simulink model "sousMarin_"  (R2021a)
settings: Solver=VariableStepAuto  StartTime=0.0  StopTime=3000  RelTol=1e-3
values from neighbouring files (symbols this model uses):
  BAT_AUTONOMY_S = BAT_AUTONOMY_H * 3600    (= 72000)    [init_values.m]
  INIT_NIV_BAT = 50    [init_values.m]
  SIMU_ACCEL = 10    [init_values.m]
  TIME_APPEL_CHARGE_S = TIME_APPEL_CHARGE_M * 60    (= 3600)    [init_values.m]
  TIME_PHOTO_S = 4    [init_values.m]
  TIME_TO_CHARGE_S = TIME_TO_CHARGE_M*60    (= 3000)    [init_values.m]
  VARIANCE_INCL_FOND = 25    [init_values.m]
  VITESSE_MAX_MS = 0.5    [init_values.m]
libraries: pid_lib x3, simulink_extras x2, simulink x1, truetime x1
settings Model: SimulationMode=accelerator  Creator=jelefl  LastModifiedBy=yamouh
settings SolverCC: AlgebraicLoopSolver=TrustRegion
settings DebuggingCC: SFMachineParentedDataDiag=warning

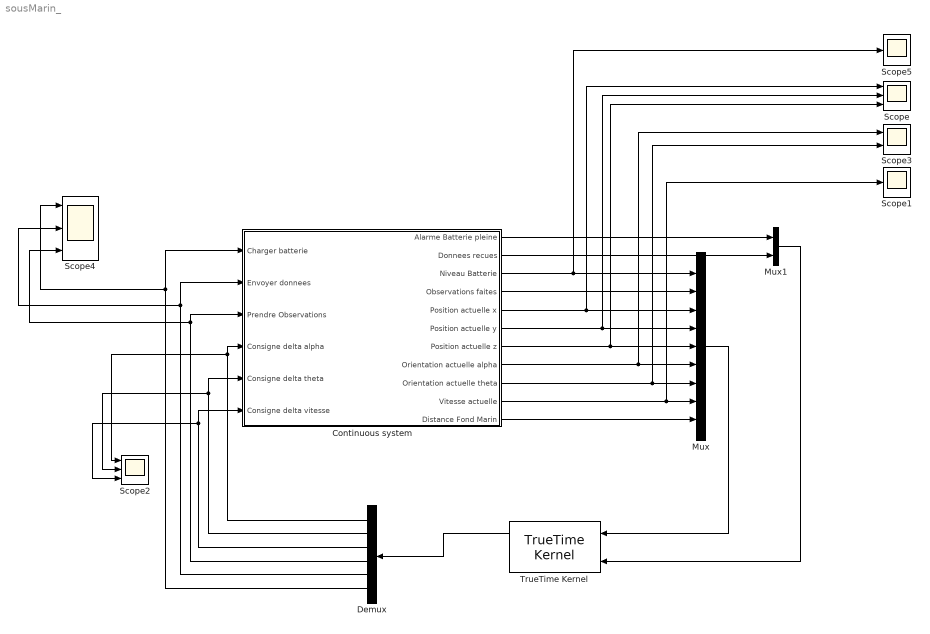
== system sousMarin_ ==
  Continuous system : Subsystem
  Demux : Demux  Outputs=6
  Mux : Mux  Inputs=9
  Mux1 : Mux  Inputs=2
  Scope : Scope  NumInputPorts=3
  Scope1 : Scope
  Scope2 : Scope  NumInputPorts=3
  Scope3 : Scope  NumInputPorts=2
  Scope4 : Scope  NumInputPorts=3
  Scope5 : Scope
  TrueTime Kernel : truetime/TrueTime Kernel  sfun=ctrlSM  args=[]  ninputsoutputs=[9 6]  ntriggers=2  trigtype=falling  nwnodenbr=[]  clockoffsetdrift=[0 0]  schedoutput=on  battery=off  poweroutput=off
  wires:
  Continuous system/3(Niveau Batterie) -> Scope5/1, Mux/1
  Continuous system/5(Position actuelle x) -> Scope/1, Mux/3
  Continuous system/6(Position actuelle y) -> Scope/2, Mux/4
  Continuous system/7(Position actuelle z) -> Scope/3, Mux/5
  Continuous system/8(Orientation actuelle alpha) -> Mux/6, Scope3/1
  Continuous system/9(Orientation actuelle theta) -> Mux/7, Scope3/2
  Mux/1 -> TrueTime Kernel/1
  TrueTime Kernel/1 -> Demux/1
  Demux/2 -> Scope2/2, Continuous system/5(Consigne delta theta)
  Demux/3 -> Scope2/3, Continuous system/6(Consigne delta vitesse)
  Demux/1 -> Scope2/1, Continuous system/4(Consigne delta alpha)
  Continuous system/10(Vitesse actuelle) -> Mux/8, Scope1/1
  Continuous system/11(Distance Fond Marin) -> Mux/9
  Continuous system/4(Observations faites) -> Mux/2
  Continuous system/1(Alarme Batterie pleine) -> Mux1/1
  Continuous system/2(Donnees recues) -> Mux1/2
  Demux/4 -> Scope4/3, Continuous system/3(Prendre Observations)
  Demux/5 -> Continuous system/2(Envoyer donnees), Scope4/2
  Demux/6 -> Continuous system/1(Charger batterie), Scope4/1
  Mux1/1 -> TrueTime Kernel/2

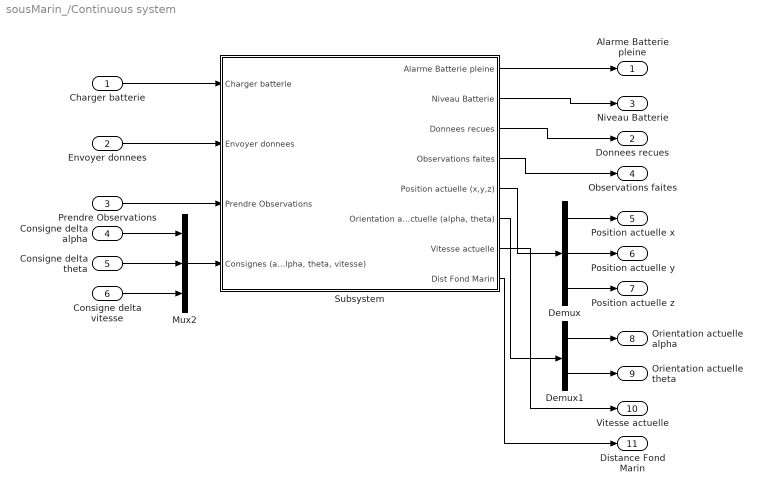
== system sousMarin_/Continuous system ==
  Charger batterie : Inport
  Envoyer donnees : Inport  Port=2
  Prendre Observations : Inport  Port=3
  Consigne delta alpha : Inport  Port=4
  Consigne delta theta : Inport  Port=5
  Consigne delta vitesse : Inport  Port=6
  Demux : Demux  Outputs=3
  Demux1 : Demux  Outputs=2
  Mux2 : Mux  Inputs=3
  Subsystem : Subsystem
  Alarme Batterie pleine : Outport  VectorParamsAs1DForOutWhenUnconnected=off
  Donnees recues : Outport  Port=2  VectorParamsAs1DForOutWhenUnconnected=off
  Niveau Batterie : Outport  Port=3  VectorParamsAs1DForOutWhenUnconnected=off
  Observations faites : Outport  Port=4  VectorParamsAs1DForOutWhenUnconnected=off
  Position actuelle x : Outport  Port=5  VectorParamsAs1DForOutWhenUnconnected=off
  Position actuelle y : Outport  Port=6  VectorParamsAs1DForOutWhenUnconnected=off
  Position actuelle z : Outport  Port=7  VectorParamsAs1DForOutWhenUnconnected=off
  Orientation actuelle alpha : Outport  Port=8  VectorParamsAs1DForOutWhenUnconnected=off
  Orientation actuelle theta : Outport  Port=9  VectorParamsAs1DForOutWhenUnconnected=off
  Vitesse actuelle : Outport  Port=10  VectorParamsAs1DForOutWhenUnconnected=off
  Distance Fond Marin : Outport  Port=11  VectorParamsAs1DForOutWhenUnconnected=off
  wires:
  Prendre Observations/1 -> Subsystem/3(Prendre Observations)
  Envoyer donnees/1 -> Subsystem/2(Envoyer donnees)
  Charger batterie/1 -> Subsystem/1(Charger batterie)
  Mux2/1 -> Subsystem/4("Consignes (alpha, theta, vitesse)")
  Consigne delta alpha/1 -> Mux2/1
  Consigne delta theta/1 -> Mux2/2
  Consigne delta vitesse/1 -> Mux2/3
  Subsystem/1(Alarme Batterie pleine) -> Alarme Batterie pleine/1
  Subsystem/2(Niveau Batterie) -> Niveau Batterie/1
  Subsystem/3(Donnees recues) -> Donnees recues/1
  Subsystem/4(Observations faites) -> Observations faites/1
  Subsystem/5(Position actuelle (x,y,z)) -> Demux/1
  Demux/1 -> Position actuelle x/1
  Demux/2 -> Position actuelle y/1
  Demux/3 -> Position actuelle z/1
  Demux1/1 -> Orientation actuelle alpha/1
  Demux1/2 -> Orientation actuelle theta/1
  Subsystem/6("Orientation actuelle (alpha, theta)") -> Demux1/1
  Subsystem/7(Vitesse actuelle) -> Vitesse actuelle/1
  Subsystem/8(Dist Fond Marin) -> Distance Fond Marin/1

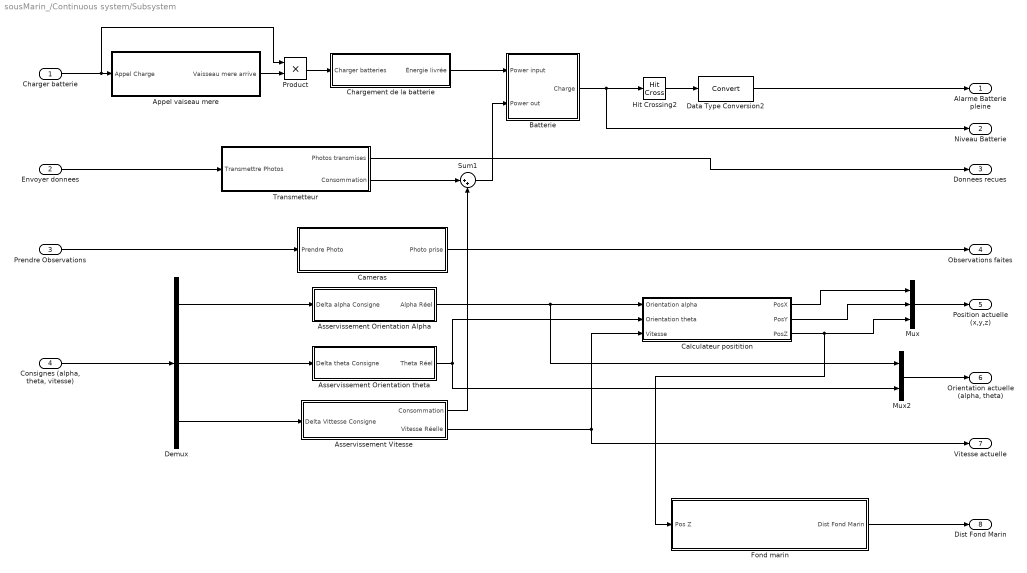
== system sousMarin_/Continuous system/Subsystem ==
  Charger batterie : Inport
  Envoyer donnees : Inport  Port=2
  Prendre Observations : Inport  Port=3
  "Consignes (alpha, theta, vitesse)" : Inport  Port=4
  Appel vaiseau mere : Subsystem
  Asservissement Orientation Alpha : Subsystem
  Asservissement Orientation theta : Subsystem
  Asservissement Vitesse : Subsystem
  Batterie : Subsystem
  Calculateur positition : Subsystem
  Cameras : Subsystem
  Chargement de la batterie : Subsystem
  Data Type Conversion2 : DataTypeConversion
  Demux : Demux  Outputs=3
  Fond marin : Subsystem
  Hit Crossing2 : HitCross  HitCrossingOffset=99.99  HitCrossingDirection=rising
  Mux : Mux  Inputs=3
  Mux2 : Mux  Inputs=2
  Product : Product
  Sum1 : Sum  Inputs=|++
  Transmetteur : Subsystem
  Alarme Batterie pleine : Outport  VectorParamsAs1DForOutWhenUnconnected=off
  Niveau Batterie : Outport  Port=2  VectorParamsAs1DForOutWhenUnconnected=off
  Donnees recues : Outport  Port=3  VectorParamsAs1DForOutWhenUnconnected=off
  Observations faites : Outport  Port=4  VectorParamsAs1DForOutWhenUnconnected=off
  Position actuelle (x,y,z) : Outport  Port=5  VectorParamsAs1DForOutWhenUnconnected=off
  "Orientation actuelle (alpha, theta)" : Outport  Port=6  VectorParamsAs1DForOutWhenUnconnected=off
  Vitesse actuelle : Outport  Port=7  VectorParamsAs1DForOutWhenUnconnected=off
  Dist Fond Marin : Outport  Port=8  VectorParamsAs1DForOutWhenUnconnected=off
  wires:
  Batterie/1(Charge) -> Niveau Batterie/1, Hit Crossing2/1
  Hit Crossing2/1 -> Data Type Conversion2/1
  Data Type Conversion2/1 -> Alarme Batterie pleine/1
  Calculateur positition/3(PosZ) -> Fond marin/1(Pos Z), Mux/3
  Prendre Observations/1 -> Cameras/1(Prendre Photo)
  Transmetteur/1(Photos transmises) -> Donnees recues/1
  Cameras/1(Photo prise) -> Observations faites/1
  Asservissement Vitesse/2(Vitesse Réelle) -> Calculateur positition/3(Vitesse), Vitesse actuelle/1
  Calculateur positition/2(PosY) -> Mux/2
  Calculateur positition/1(PosX) -> Mux/1
  Mux/1 -> Position actuelle (x,y,z)/1
  Chargement de la batterie/1(Énergie livrée) -> Batterie/1(Power input)
  Asservissement Orientation Alpha/1(Alpha Réel) -> Mux2/1, Calculateur positition/1(Orientation alpha)
  Envoyer donnees/1 -> Transmetteur/1(Transmettre Photos)
  Appel vaiseau mere/1(Vaisseau mere arrive) -> Product/2
  Product/1 -> Chargement de la batterie/1(Charger batteries)
  Charger batterie/1 -> Product/1, Appel vaiseau mere/1(Appel Charge)
  Asservissement Orientation theta/1(Theta Réel) -> Calculateur positition/2(Orientation theta), Mux2/2
  Sum1/1 -> Batterie/2(Power out)
  Transmetteur/2(Consommation) -> Sum1/1
  Asservissement Vitesse/1(Consommation) -> Sum1/2
  Demux/2 -> Asservissement Orientation theta/1(Delta theta Consigne)
  Demux/3 -> Asservissement Vitesse/1(Delta Vittesse Consigne)
  Demux/1 -> Asservissement Orientation Alpha/1(Delta alpha Consigne)
  "Consignes (alpha, theta, vitesse)"/1 -> Demux/1
  Mux2/1 -> "Orientation actuelle (alpha, theta)"/1
  Fond marin/1(Dist Fond Marin) -> Dist Fond Marin/1

== system sousMarin_/Continuous system/Subsystem/Appel vaiseau mere ==
  Appel Charge : Inport
  Vaisseau mere en deplacement : Subsystem  TreatAsAtomicUnit=on
  Vaisseau mere arrive : Outport  VectorParamsAs1DForOutWhenUnconnected=off
  wires:
  Vaisseau mere en deplacement/1(Vaisseau mere arrive) -> Vaisseau mere arrive/1
  Appel Charge/1 -> Vaisseau mere en deplacement/Reset

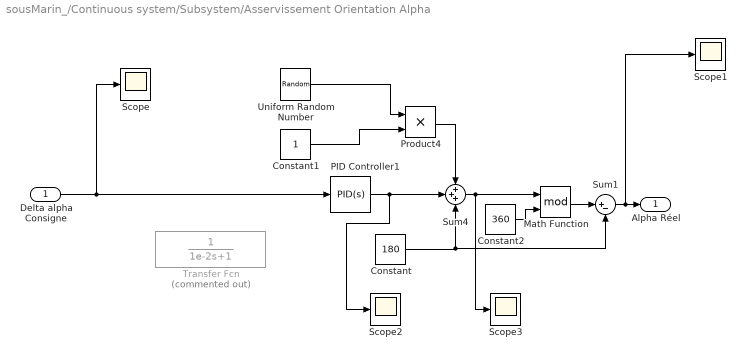
== system sousMarin_/Continuous system/Subsystem/Asservissement Orientation Alpha ==
  Delta alpha Consigne : Inport
  Constant : Constant  Value=180
  Constant1 : Constant
  Constant2 : Constant  Value=360
  Math Function : Math  Operator=mod  SaturateOnIntegerOverflow=on
  PID Controller1 : pid_lib/PID Controller  Controller=PID  Form=Parallel  TimeDomain=Continuous-time  UseExternalTs=off  SampleTime=-1  IntegratorMethod=Forward Euler  FilterMethod=Forward Euler  ControllerParametersSource=internal  P=.1  I=5  D=0  UseFilter=on  N=0.1  TunerSelectOption=Transfer Function Based (PID Tuner App)  InitialConditionSource=internal  InitialConditionForIntegrator=0  InitialConditionForFilter=0  DifferentiatorICPrevScaledInput=0  ExternalReset=none  TrackingMode=off  Kt=1  LimitOutput=off  SatLimitsSource=internal  UpperSaturationLimit=inf  LowerSaturationLimit=-inf  LinearizeAsGain=on  AntiWindupMode=none  Kb=1  POutMin=[]  POutMax=[]  IOutMin=[]  IOutMax=[]  DOutMin=[]  DOutMax=[]  NOutMin=[]  NOutMax=[]  SumOutMin=[]  SumOutMax=[]  SaturationOutMin=[]  SaturationOutMax=[]  PParamMin=[]  PParamMax=[]  IParamMin=[]  IParamMax=[]  DParamMin=[]  DParamMax=[]  NParamMin=[]  NParamMax=[]  KbParamMin=[]  KbParamMax=[]  KtParamMin=[]  KtParamMax=[]  KbOutMin=[]  KbOutMax=[]  KtOutMin=[]  KtOutMax=[]  IntegratorOutMin=[]  IntegratorOutMax=[]  FilterOutMin=[]  FilterOutMax=[]  SumI1OutMin=[]  SumI1OutMax=[]  SumI2OutMin=[]  SumI2OutMax=[]  SumI3OutMin=[]  SumI3OutMax=[]  SumI4OutMin=[]  SumI4OutMax=[]  SumDOutMin=[]  SumDOutMax=[]  DifferentiatorOutMin=[]  DifferentiatorOutMax=[]  FilterDiffOutCoefMin=[]  FilterDiffOutCoefMax=[]  ReciprocalOutMin=[]  ReciprocalOutMax=[]  SumDenOutMin=[]  SumDenOutMax=[]  SumNumOutMin=[]  SumNumOutMax=[]  DivideOutMin=[]  DivideOutMax=[]  UdiffTsProdOutMin=[]  UdiffTsProdOutMax=[]  NTsProdOutMin=[]  NTsProdOutMax=[]  UintegralTsProdOutMin=[]  UintegralTsProdOutMax=[]  UngainTsProdOutMin=[]  UngainTsProdOutMax=[]  IntegratorContinuousStateAttributes=''  IntegratorStateMustResolveToSignalObject=off  IntegratorRTWStateStorageClass=Auto  FilterContinuousStateAttributes=''  FilterStateMustResolveToSignalObject=off  FilterRTWStateStorageClass=Auto  ParallelPVariant=InternalParameters  IdealPVariant=Disabled  IVariant=InternalParameters  DVariant=InternalParameters  IntegratorVariant=Continuous  SatVariant=Disabled  AWVariant=Passthrough  PCopyVariant=Disabled  TRVariant=Disabled  FdbkBlocksVariant=Forward  IdealPFdbkVariant=Disabled  SatFdbkVariant=Disabled  DerivativeFilterVariant=ContFilter  NVariant=InternalParameters  NCopyVariant=Disabled  FilterICVariant=InternalICsFilter  IntegratorICVariant=InternalICs  ExternalResetVariant=Disabled  TRSumVariant=Passthrough  SumFdbkVariant=Disabled  SumVariant=Sum_PID  TsampFilterVariant=InternalTs  TsampNgainVariant=Passthrough  TsampIntegralVariant=Passthrough  ExternalSaturationOutDataTypeStr=Inherit: Same as second input
  Product4 : Product
  Scope{,1..3} (4 alike) : Scope
  Sum1 : Sum  Inputs=|+-
  Sum4 : Sum  Inputs=+++
  Transfer Fcn : TransferFcn  Commented=on  Denominator=[1e-2 1]
  Uniform Random Number : UniformRandomNumber  SampleTime=0.1
  Alpha Réel : Outport  VectorParamsAs1DForOutWhenUnconnected=off
  wires:
  Product4/1 -> Sum4/1
  Uniform Random Number/1 -> Product4/1
  Constant1/1 -> Product4/2
  PID Controller1/1 -> Scope2/1, Sum4/2
  Delta alpha Consigne/1 -> PID Controller1/1, Scope/1
  Constant/1 -> Sum4/3, Sum1/2
  Math Function/1 -> Sum1/1
  Constant2/1 -> Math Function/2
  Sum1/1 -> Scope1/1, Alpha Réel/1
  Sum4/1 -> Scope3/1, Math Function/1

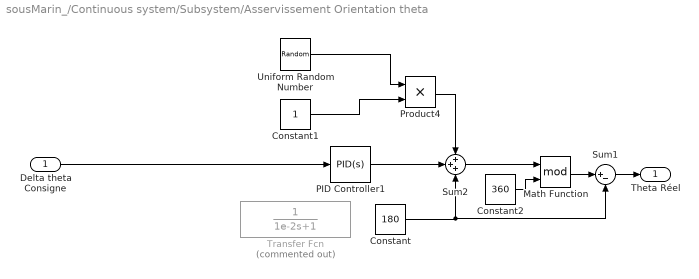
== system sousMarin_/Continuous system/Subsystem/Asservissement Orientation theta ==
  Delta theta Consigne : Inport
  Constant : Constant  Value=180
  Constant1 : Constant
  Constant2 : Constant  Value=360
  Math Function : Math  Operator=mod  SaturateOnIntegerOverflow=on
  PID Controller1 : pid_lib/PID Controller  Controller=PID  Form=Parallel  TimeDomain=Continuous-time  UseExternalTs=off  SampleTime=-1  IntegratorMethod=Forward Euler  FilterMethod=Forward Euler  ControllerParametersSource=internal  P=.1  I=5  D=0  UseFilter=on  N=0.1  TunerSelectOption=Transfer Function Based (PID Tuner App)  InitialConditionSource=internal  InitialConditionForIntegrator=0  InitialConditionForFilter=0  DifferentiatorICPrevScaledInput=0  ExternalReset=none  TrackingMode=off  Kt=1  LimitOutput=off  SatLimitsSource=internal  UpperSaturationLimit=inf  LowerSaturationLimit=-inf  LinearizeAsGain=on  AntiWindupMode=none  Kb=1  POutMin=[]  POutMax=[]  IOutMin=[]  IOutMax=[]  DOutMin=[]  DOutMax=[]  NOutMin=[]  NOutMax=[]  SumOutMin=[]  SumOutMax=[]  SaturationOutMin=[]  SaturationOutMax=[]  PParamMin=[]  PParamMax=[]  IParamMin=[]  IParamMax=[]  DParamMin=[]  DParamMax=[]  NParamMin=[]  NParamMax=[]  KbParamMin=[]  KbParamMax=[]  KtParamMin=[]  KtParamMax=[]  KbOutMin=[]  KbOutMax=[]  KtOutMin=[]  KtOutMax=[]  IntegratorOutMin=[]  IntegratorOutMax=[]  FilterOutMin=[]  FilterOutMax=[]  SumI1OutMin=[]  SumI1OutMax=[]  SumI2OutMin=[]  SumI2OutMax=[]  SumI3OutMin=[]  SumI3OutMax=[]  SumI4OutMin=[]  SumI4OutMax=[]  SumDOutMin=[]  SumDOutMax=[]  DifferentiatorOutMin=[]  DifferentiatorOutMax=[]  FilterDiffOutCoefMin=[]  FilterDiffOutCoefMax=[]  ReciprocalOutMin=[]  ReciprocalOutMax=[]  SumDenOutMin=[]  SumDenOutMax=[]  SumNumOutMin=[]  SumNumOutMax=[]  DivideOutMin=[]  DivideOutMax=[]  UdiffTsProdOutMin=[]  UdiffTsProdOutMax=[]  NTsProdOutMin=[]  NTsProdOutMax=[]  UintegralTsProdOutMin=[]  UintegralTsProdOutMax=[]  UngainTsProdOutMin=[]  UngainTsProdOutMax=[]  IntegratorContinuousStateAttributes=''  IntegratorStateMustResolveToSignalObject=off  IntegratorRTWStateStorageClass=Auto  FilterContinuousStateAttributes=''  FilterStateMustResolveToSignalObject=off  FilterRTWStateStorageClass=Auto  ParallelPVariant=InternalParameters  IdealPVariant=Disabled  IVariant=InternalParameters  DVariant=InternalParameters  IntegratorVariant=Continuous  SatVariant=Disabled  AWVariant=Passthrough  PCopyVariant=Disabled  TRVariant=Disabled  FdbkBlocksVariant=Forward  IdealPFdbkVariant=Disabled  SatFdbkVariant=Disabled  DerivativeFilterVariant=ContFilter  NVariant=InternalParameters  NCopyVariant=Disabled  FilterICVariant=InternalICsFilter  IntegratorICVariant=InternalICs  ExternalResetVariant=Disabled  TRSumVariant=Passthrough  SumFdbkVariant=Disabled  SumVariant=Sum_PID  TsampFilterVariant=InternalTs  TsampNgainVariant=Passthrough  TsampIntegralVariant=Passthrough  ExternalSaturationOutDataTypeStr=Inherit: Same as second input
  Product4 : Product
  Sum1 : Sum  Inputs=|+-
  Sum2 : Sum  Inputs=+++
  Transfer Fcn : TransferFcn  Commented=on  Denominator=[1e-2 1]
  Uniform Random Number : UniformRandomNumber  SampleTime=0.1
  Theta Réel : Outport  VectorParamsAs1DForOutWhenUnconnected=off
  wires:
  Product4/1 -> Sum2/1
  Uniform Random Number/1 -> Product4/1
  Constant1/1 -> Product4/2
  PID Controller1/1 -> Sum2/2
  Delta theta Consigne/1 -> PID Controller1/1
  Sum1/1 -> Theta Réel/1
  Constant/1 -> Sum2/3, Sum1/2
  Constant2/1 -> Math Function/2
  Math Function/1 -> Sum1/1
  Sum2/1 -> Math Function/1

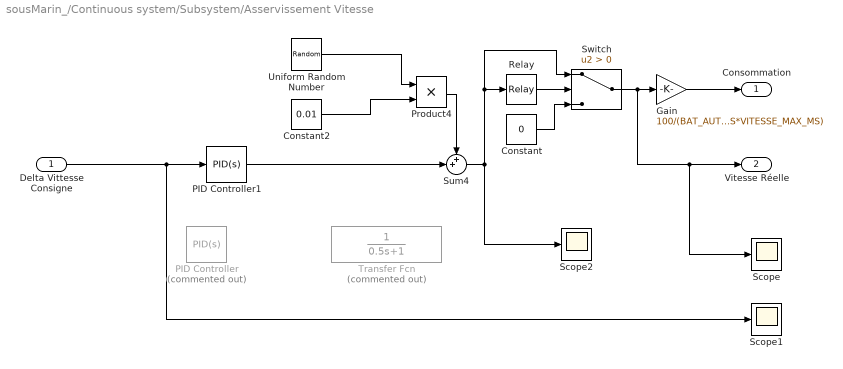
== system sousMarin_/Continuous system/Subsystem/Asservissement Vitesse ==
  Delta Vittesse Consigne : Inport
  Constant : Constant  Value=0
  Constant2 : Constant  Value=0.01
  Gain : Gain  Gain=100/(BAT_AUTONOMY_S*VITESSE_MAX_MS)
  PID Controller : simulink/Continuous/PID Controller  Commented=on  Controller=PID  Form=Parallel  TimeDomain=Continuous-time  UseExternalTs=off  SampleTime=-1  IntegratorMethod=Forward Euler  FilterMethod=Forward Euler  ControllerParametersSource=internal  P=1  I=1  D=0  UseFilter=on  N=100  TunerSelectOption=Transfer Function Based (PID Tuner App)  InitialConditionSource=internal  InitialConditionForIntegrator=0  InitialConditionForFilter=0  DifferentiatorICPrevScaledInput=0  ExternalReset=none  TrackingMode=off  Kt=1  LimitOutput=off  UpperSaturationLimit=inf  LowerSaturationLimit=-inf  LinearizeAsGain=on  AntiWindupMode=none  Kb=1  POutMin=[]  POutMax=[]  IOutMin=[]  IOutMax=[]  DOutMin=[]  DOutMax=[]  NOutMin=[]  NOutMax=[]  SumOutMin=[]  SumOutMax=[]  SaturationOutMin=[]  SaturationOutMax=[]  PParamMin=[]  PParamMax=[]  IParamMin=[]  IParamMax=[]  DParamMin=[]  DParamMax=[]  NParamMin=[]  NParamMax=[]  KbParamMin=[]  KbParamMax=[]  KtParamMin=[]  KtParamMax=[]  KbOutMin=[]  KbOutMax=[]  KtOutMin=[]  KtOutMax=[]  IntegratorOutMin=[]  IntegratorOutMax=[]  FilterOutMin=[]  FilterOutMax=[]  SumI1OutMin=[]  SumI1OutMax=[]  SumI2OutMin=[]  SumI2OutMax=[]  SumI3OutMin=[]  SumI3OutMax=[]  SumI4OutMin=[]  SumI4OutMax=[]  SumDOutMin=[]  SumDOutMax=[]  DifferentiatorOutMin=[]  DifferentiatorOutMax=[]  FilterDiffOutCoefMin=[]  FilterDiffOutCoefMax=[]  ReciprocalOutMin=[]  ReciprocalOutMax=[]  SumDenOutMin=[]  SumDenOutMax=[]  SumNumOutMin=[]  SumNumOutMax=[]  DivideOutMin=[]  DivideOutMax=[]  UdiffTsProdOutMin=[]  UdiffTsProdOutMax=[]  NTsProdOutMin=[]  NTsProdOutMax=[]  UintegralTsProdOutMin=[]  UintegralTsProdOutMax=[]  UngainTsProdOutMin=[]  UngainTsProdOutMax=[]  IntegratorContinuousStateAttributes=''  IntegratorStateMustResolveToSignalObject=off  IntegratorRTWStateStorageClass=Auto  FilterContinuousStateAttributes=''  FilterStateMustResolveToSignalObject=off  FilterRTWStateStorageClass=Auto  ParallelPVariant=InternalParameters  IdealPVariant=Disabled  IVariant=InternalParameters  DVariant=InternalParameters  IntegratorVariant=Continuous  SatVariant=Disabled  AWVariant=Passthrough  PCopyVariant=Disabled  TRVariant=Disabled  FdbkBlocksVariant=Forward  IdealPFdbkVariant=Disabled  SatFdbkVariant=Disabled  DerivativeFilterVariant=ContFilter  NVariant=InternalParameters  NCopyVariant=Disabled  FilterICVariant=InternalICsFilter  IntegratorICVariant=InternalICs  ExternalResetVariant=Disabled  TRSumVariant=Passthrough  SumFdbkVariant=Disabled  SumVariant=Sum_PID  TsampFilterVariant=InternalTs  TsampNgainVariant=Passthrough  TsampIntegralVariant=Passthrough
  PID Controller1 : pid_lib/PID Controller  Controller=PID  Form=Parallel  TimeDomain=Continuous-time  UseExternalTs=off  SampleTime=-1  IntegratorMethod=Forward Euler  FilterMethod=Forward Euler  ControllerParametersSource=internal  P=.1  I=5  D=0  UseFilter=on  N=0.1  TunerSelectOption=Transfer Function Based (PID Tuner App)  InitialConditionSource=internal  InitialConditionForIntegrator=0  InitialConditionForFilter=0  DifferentiatorICPrevScaledInput=0  ExternalReset=none  TrackingMode=off  Kt=1  LimitOutput=off  SatLimitsSource=internal  UpperSaturationLimit=inf  LowerSaturationLimit=-inf  LinearizeAsGain=on  AntiWindupMode=none  Kb=1  POutMin=[]  POutMax=[]  IOutMin=[]  IOutMax=[]  DOutMin=[]  DOutMax=[]  NOutMin=[]  NOutMax=[]  SumOutMin=[]  SumOutMax=[]  SaturationOutMin=[]  SaturationOutMax=[]  PParamMin=[]  PParamMax=[]  IParamMin=[]  IParamMax=[]  DParamMin=[]  DParamMax=[]  NParamMin=[]  NParamMax=[]  KbParamMin=[]  KbParamMax=[]  KtParamMin=[]  KtParamMax=[]  KbOutMin=[]  KbOutMax=[]  KtOutMin=[]  KtOutMax=[]  IntegratorOutMin=[]  IntegratorOutMax=[]  FilterOutMin=[]  FilterOutMax=[]  SumI1OutMin=[]  SumI1OutMax=[]  SumI2OutMin=[]  SumI2OutMax=[]  SumI3OutMin=[]  SumI3OutMax=[]  SumI4OutMin=[]  SumI4OutMax=[]  SumDOutMin=[]  SumDOutMax=[]  DifferentiatorOutMin=[]  DifferentiatorOutMax=[]  FilterDiffOutCoefMin=[]  FilterDiffOutCoefMax=[]  ReciprocalOutMin=[]  ReciprocalOutMax=[]  SumDenOutMin=[]  SumDenOutMax=[]  SumNumOutMin=[]  SumNumOutMax=[]  DivideOutMin=[]  DivideOutMax=[]  UdiffTsProdOutMin=[]  UdiffTsProdOutMax=[]  NTsProdOutMin=[]  NTsProdOutMax=[]  UintegralTsProdOutMin=[]  UintegralTsProdOutMax=[]  UngainTsProdOutMin=[]  UngainTsProdOutMax=[]  IntegratorContinuousStateAttributes=''  IntegratorStateMustResolveToSignalObject=off  IntegratorRTWStateStorageClass=Auto  FilterContinuousStateAttributes=''  FilterStateMustResolveToSignalObject=off  FilterRTWStateStorageClass=Auto  ParallelPVariant=InternalParameters  IdealPVariant=Disabled  IVariant=InternalParameters  DVariant=InternalParameters  IntegratorVariant=Continuous  SatVariant=Disabled  AWVariant=Passthrough  PCopyVariant=Disabled  TRVariant=Disabled  FdbkBlocksVariant=Forward  IdealPFdbkVariant=Disabled  SatFdbkVariant=Disabled  DerivativeFilterVariant=ContFilter  NVariant=InternalParameters  NCopyVariant=Disabled  FilterICVariant=InternalICsFilter  IntegratorICVariant=InternalICs  ExternalResetVariant=Disabled  TRSumVariant=Passthrough  SumFdbkVariant=Disabled  SumVariant=Sum_PID  TsampFilterVariant=InternalTs  TsampNgainVariant=Passthrough  TsampIntegralVariant=Passthrough  ExternalSaturationOutDataTypeStr=Inherit: Same as second input
  Product4 : Product
  Relay : Relay  OnSwitchValue=0.011  OffSwitchValue=0.01
  Scope : Scope
  Scope1 : Scope
  Scope2 : Scope
  Sum4 : Sum  Inputs=++|
  Switch : Switch  Criteria=u2 > Threshold
  Transfer Fcn : TransferFcn  Commented=on  Denominator=[0.5 1]
  Uniform Random Number : UniformRandomNumber  SampleTime=0.1
  Consommation : Outport  VectorParamsAs1DForOutWhenUnconnected=off
  Vitesse Réelle : Outport  Port=2  VectorParamsAs1DForOutWhenUnconnected=off
  wires:
  Sum4/1 -> Switch/1, Relay/1, Scope2/1
  Relay/1 -> Switch/2
  Gain/1 -> Consommation/1
  Constant/1 -> Switch/3
  Uniform Random Number/1 -> Product4/1
  Constant2/1 -> Product4/2
  Product4/1 -> Sum4/1
  Delta Vittesse Consigne/1 -> Scope1/1, PID Controller1/1
  PID Controller1/1 -> Sum4/2
  Switch/1 -> Scope/1, Vitesse Réelle/1, Gain/1

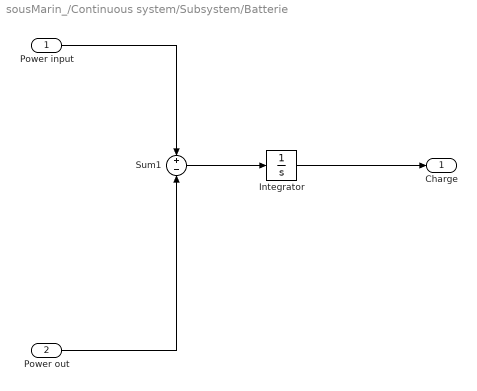
== system sousMarin_/Continuous system/Subsystem/Batterie ==
  Power input : Inport
  Power out : Inport  Port=2
  Integrator : Integrator  InitialCondition=INIT_NIV_BAT  LimitOutput=on  UpperSaturationLimit=100  LowerSaturationLimit=0
  Sum1 : Sum  Inputs=+-
  Charge : Outport  VectorParamsAs1DForOutWhenUnconnected=off
  wires:
  Sum1/1 -> Integrator/1
  Power input/1 -> Sum1/1
  Power out/1 -> Sum1/2
  Integrator/1 -> Charge/1

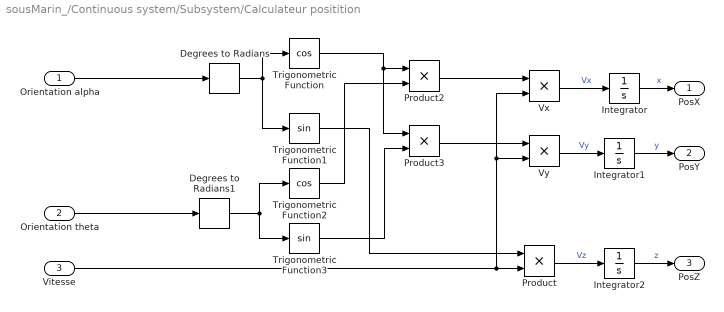
== system sousMarin_/Continuous system/Subsystem/Calculateur positition ==
  Orientation alpha : Inport
  Orientation theta : Inport  Port=2
  Vitesse : Inport  Port=3
  Degrees to Radians : simulink_extras/Transformations/Degrees to Radians
  Degrees to Radians1 : simulink_extras/Transformations/Degrees to Radians
  Integrator : Integrator
  Integrator1 : Integrator
  Integrator2 : Integrator  LimitOutput=on  UpperSaturationLimit=0
  Product : Product
  Product2 : Product
  Product3 : Product
  Trigonometric Function : Trigonometry  Operator=cos
  Trigonometric Function1 : Trigonometry
  Trigonometric Function2 : Trigonometry  Operator=cos
  Trigonometric Function3 : Trigonometry
  Vx : Product
  Vy : Product
  PosX : Outport  VectorParamsAs1DForOutWhenUnconnected=off
  PosY : Outport  Port=2  VectorParamsAs1DForOutWhenUnconnected=off
  PosZ : Outport  Port=3  VectorParamsAs1DForOutWhenUnconnected=off
  wires:
  Trigonometric Function3/1 -> Product3/2
  Product3/1 -> Vy/1
  Vx/1 -> Integrator/1  "Vx"
  Vitesse/1 -> Vy/2, Vx/2, Product/2
  Product2/1 -> Vx/1
  Product/1 -> Integrator2/1  "Vz"
  Integrator1/1 -> PosY/1  "y"
  Degrees to Radians1/1 -> Trigonometric Function2/1, Trigonometric Function3/1
  Orientation theta/1 -> Degrees to Radians1/1
  Orientation alpha/1 -> Degrees to Radians/1
  Degrees to Radians/1 -> Trigonometric Function1/1, Trigonometric Function/1
  Trigonometric Function/1 -> Product2/1, Product3/1
  Trigonometric Function1/1 -> Product/1
  Vy/1 -> Integrator1/1  "Vy"
  Integrator/1 -> PosX/1  "x"
  Trigonometric Function2/1 -> Product2/2
  Integrator2/1 -> PosZ/1  "z"

== system sousMarin_/Continuous system/Subsystem/Cameras ==
  Prendre Photo : Inport
  Prise photo : Subsystem  TreatAsAtomicUnit=on
  Photo prise : Outport  VectorParamsAs1DForOutWhenUnconnected=off
  wires:
  Prise photo/1(Out1) -> Photo prise/1
  Prendre Photo/1 -> Prise photo/Reset

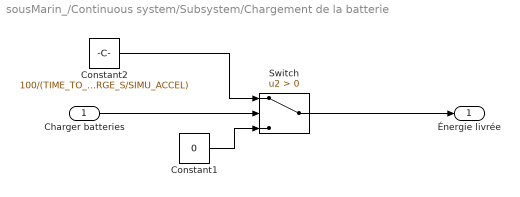
== system sousMarin_/Continuous system/Subsystem/Chargement de la batterie ==
  Charger batteries : Inport
  Constant1 : Constant  Value=0
  Constant2 : Constant  Value=100/(TIME_TO_CHARGE_S/SIMU_ACCEL)
  Switch : Switch  Criteria=u2 > Threshold
  Énergie livrée : Outport  VectorParamsAs1DForOutWhenUnconnected=off
  wires:
  Charger batteries/1 -> Switch/2
  Constant1/1 -> Switch/3
  Switch/1 -> Énergie livrée/1
  Constant2/1 -> Switch/1

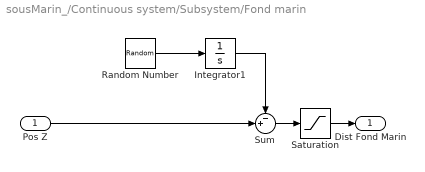
== system sousMarin_/Continuous system/Subsystem/Fond marin ==
  Pos Z : Inport
  Integrator1 : Integrator  InitialCondition=-1000  LimitOutput=on  UpperSaturationLimit=-800  LowerSaturationLimit=-1200
  Random Number : RandomNumber  Variance=VARIANCE_INCL_FOND  SampleTime=10
  Saturation : Saturate  UpperLimit=1200  LowerLimit=5
  Sum : Sum  Inputs=-+|
  Dist Fond Marin : Outport
  wires:
  Random Number/1 -> Integrator1/1
  Integrator1/1 -> Sum/1
  Pos Z/1 -> Sum/2
  Sum/1 -> Saturation/1
  Saturation/1 -> Dist Fond Marin/1

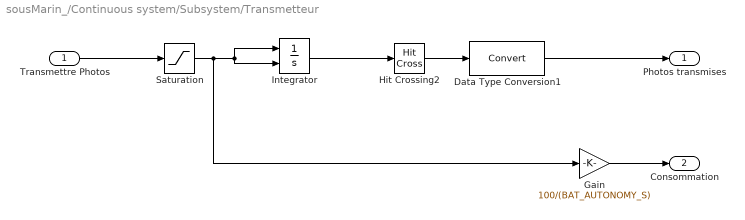
== system sousMarin_/Continuous system/Subsystem/Transmetteur ==
  Transmettre Photos : Inport
  Data Type Conversion1 : DataTypeConversion
  Gain : Gain  Gain=100/(BAT_AUTONOMY_S)
  Hit Crossing2 : HitCross  HitCrossingOffset=TIME_TRANSM_S  HitCrossingDirection=rising
  Integrator : Integrator  ExternalReset=rising
  Saturation : Saturate  UpperLimit=1  LowerLimit=0
  Photos transmises : Outport  VectorParamsAs1DForOutWhenUnconnected=off
  Consommation : Outport  Port=2  VectorParamsAs1DForOutWhenUnconnected=off
  wires:
  Data Type Conversion1/1 -> Photos transmises/1
  Integrator/1 -> Hit Crossing2/1
  Hit Crossing2/1 -> Data Type Conversion1/1
  Transmettre Photos/1 -> Saturation/1
  Saturation/1 -> Gain/1, Integrator/2, Integrator/1
  Gain/1 -> Consommation/1

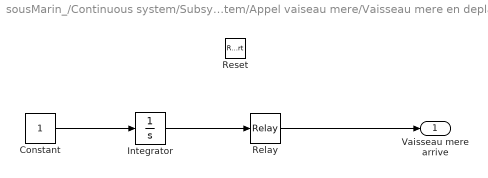
== system sousMarin_/Continuous system/Subsystem/Appel vaiseau mere/Vaisseau mere en deplacement ==
  Reset : ResetPort  DisableCoverage=on
  Constant : Constant
  Integrator : Integrator
  Relay : Relay  OnSwitchValue=TIME_APPEL_CHARGE_S/SIMU_ACCEL  OffSwitchValue=0
  Vaisseau mere arrive : Outport  VectorParamsAs1DForOutWhenUnconnected=off
  wires:
  Integrator/1 -> Relay/1
  Constant/1 -> Integrator/1
  Relay/1 -> Vaisseau mere arrive/1

== system sousMarin_/Continuous system/Subsystem/Cameras/Prise photo ==
  Reset : ResetPort  DisableCoverage=on
  Constant : Constant
  Integrator : Integrator
  Relay : Relay  OnSwitchValue=TIME_PHOTO_S  OffSwitchValue=0
  Out1 : Outport  VectorParamsAs1DForOutWhenUnconnected=off
  wires:
  Integrator/1 -> Relay/1
  Constant/1 -> Integrator/1
  Relay/1 -> Out1/1
